simulink model "SNN_circuit11"  (R2021a)
settings: Solver=FixedStepAuto  StartTime=0.0  StopTime=50  FixedStep=1e-3  RelTol=1e-3
values from neighbouring files (symbols this model uses):
  l = 100e-6    (= 0.0001)    [SNN_run_main11.m]    (also in SNN_run_main22.m; SNN_run_main33.m)
libraries: fl_lib x57, nesl_utility x20, ee_lib x5
(part 1 of 2)
settings Model: Creator=yeeyoung  LastModifiedBy=yangy
settings SolverCC: ZeroCrossAlgorithm=Adaptive  AlgebraicLoopSolver=TrustRegion  DecoupledContinuousIntegration=on  MinimalZcImpactIntegration=on
settings DebuggingCC: SFMachineParentedDataDiag=warning
settings SimscapeCC: SimscapeLogType=all  SimscapeLogSimulationStatistics=on  SimscapeLogName=SNN_circuit1  SimscapeLogDataHistory=35000

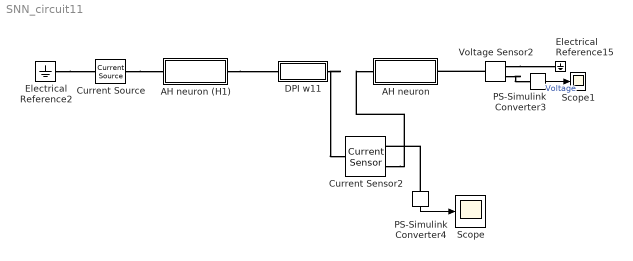
== system SNN_circuit11 ==
  AH neuron : Subsystem
  AH neuron (H1) : Subsystem
  Current Sensor2 : fl_lib/Electrical/Electrical Sensors/Current Sensor
  Current Source : ee_lib/Sources/Current Source  dc_current=Iin1 nA  ac_current=0 nA  ac_shift=0 rad  ac_frequency=60 Hz  noise_mode=0  PSD=0 A^2/Hz  repeatability=1  auto_seed=703320810  user_seed=0  sample_time=1e-3 s  i_specify=off  i_priority=None  i=0 A  i_nominal_specify=off  i_nominal_unit=A  i_nominal_value=1  v_specify=off  v_priority=None  v=0 V  v_nominal_specify=off  v_nominal_unit=V  v_nominal_value=1
      settings: SourceProductBaseCode=PS
  DPI w11 : Subsystem
  Electrical Reference15 : fl_lib/Electrical/Electrical Elements/Electrical Reference
  Electrical Reference2 : fl_lib/Electrical/Electrical Elements/Electrical Reference
  PS-Simulink Converter3 : nesl_utility/PS-Simulink Converter  PhysicalDomain=network_engine_domain  SubClassName=ps_output  LeftPortType=input  RightPortType=output  PseudoPeriodic=off  Frequencies=[]  Unit=1  AffineConversion=off
      settings: SourceProductBaseCode=PW,SS
  PS-Simulink Converter4 : nesl_utility/PS-Simulink Converter  PhysicalDomain=network_engine_domain  SubClassName=ps_output  LeftPortType=input  RightPortType=output  PseudoPeriodic=off  Frequencies=[]  Unit=1  AffineConversion=off
      settings: SourceProductBaseCode=PW,SS
  Scope : Scope
  Scope1 : Scope
  Voltage Sensor2 : fl_lib/Electrical/Electrical Sensors/Voltage Sensor
  wires:
  PS-Simulink Converter3/1 -> Scope1/1  "Voltage"
  PS-Simulink Converter4/1 -> Scope/1
  connections:
  AH neuron (H1)/RConn1 -- DPI w11/LConn1
  Voltage Sensor2/LConn1 -- AH neuron/RConn1
  Current Source/LConn1 -- AH neuron (H1)/LConn1
  Voltage Sensor2/RConn2 -- Electrical Reference15/LConn1
  Voltage Sensor2/RConn1 -- PS-Simulink Converter3/LConn1
  Electrical Reference2/LConn1 -- Current Source/RConn1
  PS-Simulink Converter4/LConn1 -- Current Sensor2/RConn1
  DPI w11/RConn1 -- Current Sensor2/LConn1
  Current Sensor2/RConn2 -- AH neuron/LConn1

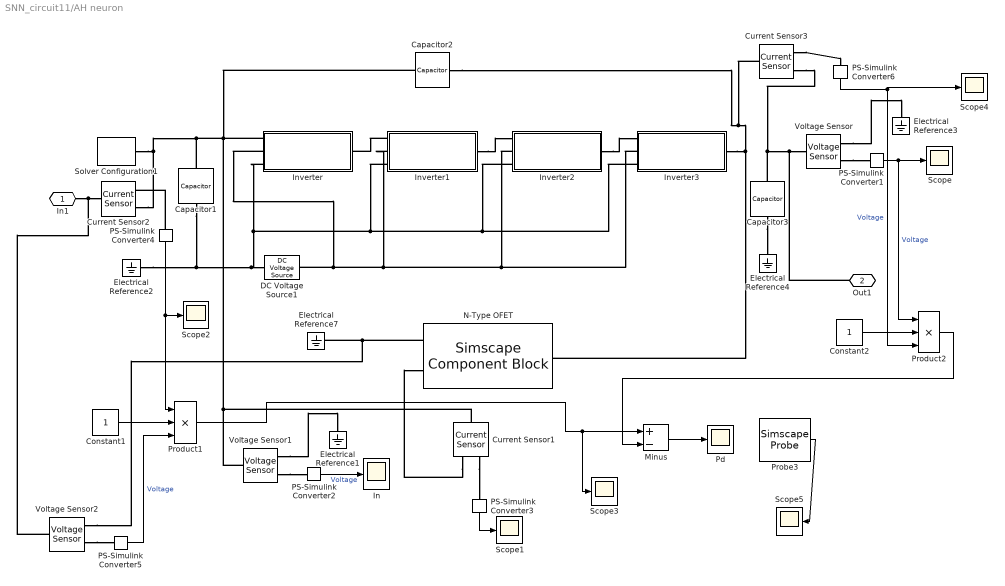
== system SNN_circuit11/AH neuron ==
  Capacitor1 : ee_lib/Passive/Capacitor  cap_option=0  c=Cmem nF  Cvec=[1e-05, 1e-06] F  Vvec=[0, 10] V  CV_table_symmetry=1  f_vec=[1, 10] kHz  DFext_vec=[.8, 1.2]  C_tol=5  enable_C_tol=0  tol_distribution=1  nSigma=4  r=1e-6 Ohm  g=0 1/Ohm  averaging_period=0 s  enable_operating_limits=0  operating_limit_action=2  max_working_voltage_range=[-25, 25] V  power_rating=1 W  enable_faults=0  fault_action=1  Cscale_faulted=100  R_faulted=1e-3 Ohm  G_faulted=0 1/Ohm  tau_fault=1e-3 s  enable_temporal_fault=0  t_fault=1 s  enable_behavioral_fault=0  max_permissible_voltage_range=[-100, 100] V  t_fail_on_voltage=1 s  i_specify=off  i_priority=None  i=0 A  i_nominal_specify=off  i_nominal_unit=A  i_nominal_value=1  v_specify=off  v_priority=None  v=0 V  v_nominal_specify=off  v_nominal_unit=V  v_nominal_value=1  vc_specify=off  vc_priority=High  vc=0 V  vc_nominal_specify=off  vc_nominal_unit=V  vc_nominal_value=1
  Capacitor2 : ee_lib/Passive/Capacitor  cap_option=0  c=Cfb nF  Cvec=[1e-05, 1e-06] F  Vvec=[0, 10] V  CV_table_symmetry=1  f_vec=[1, 10] kHz  DFext_vec=[.8, 1.2]  C_tol=5  enable_C_tol=0  tol_distribution=1  nSigma=4  r=1e-6 Ohm  g=0 1/Ohm  averaging_period=0 s  enable_operating_limits=0  operating_limit_action=2  max_working_voltage_range=[-25, 25] V  power_rating=1 W  enable_faults=0  fault_action=1  Cscale_faulted=100  R_faulted=1e-3 Ohm  G_faulted=0 1/Ohm  tau_fault=1e-3 s  enable_temporal_fault=0  t_fault=1 s  enable_behavioral_fault=0  max_permissible_voltage_range=[-100, 100] V  t_fail_on_voltage=1 s  i_specify=off  i_priority=None  i=0 A  i_nominal_specify=off  i_nominal_unit=A  i_nominal_value=1  v_specify=off  v_priority=None  v=0 V  v_nominal_specify=off  v_nominal_unit=V  v_nominal_value=1  vc_specify=off  vc_priority=High  vc=0 V  vc_nominal_specify=off  vc_nominal_unit=V  vc_nominal_value=1
  Capacitor3 : ee_lib/Passive/Capacitor  cap_option=0  c=Cload nF  Cvec=[1e-05, 1e-06] F  Vvec=[0, 10] V  CV_table_symmetry=1  f_vec=[1, 10] kHz  DFext_vec=[.8, 1.2]  C_tol=5  enable_C_tol=0  tol_distribution=1  nSigma=4  r=1e-6 Ohm  g=0 1/Ohm  averaging_period=0 s  enable_operating_limits=0  operating_limit_action=2  max_working_voltage_range=[-25, 25] V  power_rating=1 W  enable_faults=0  fault_action=1  Cscale_faulted=100  R_faulted=1e-3 Ohm  G_faulted=0 1/Ohm  tau_fault=1e-3 s  enable_temporal_fault=0  t_fault=1 s  enable_behavioral_fault=0  max_permissible_voltage_range=[-100, 100] V  t_fail_on_voltage=1 s  i_specify=off  i_priority=None  i=0 A  i_nominal_specify=off  i_nominal_unit=A  i_nominal_value=1  v_specify=off  v_priority=None  v=0 V  v_nominal_specify=off  v_nominal_unit=V  v_nominal_value=1  vc_specify=off  vc_priority=High  vc=0 V  vc_nominal_specify=off  vc_nominal_unit=V  vc_nominal_value=1
  Constant1 : Constant
  Constant2 : Constant
  Current Sensor1 : fl_lib/Electrical/Electrical Sensors/Current Sensor
  Current Sensor2 : fl_lib/Electrical/Electrical Sensors/Current Sensor
  Current Sensor3 : fl_lib/Electrical/Electrical Sensors/Current Sensor
  DC Voltage Source1 : fl_lib/Electrical/Electrical Sources/DC Voltage Source  v0=Vdd_soma V
  Electrical Reference{1..4,7} (5 alike) : fl_lib/Electrical/Electrical Elements/Electrical Reference
  In : Scope
  Inverter : Subsystem
  Inverter1 : Subsystem
  Inverter2 : Subsystem
  Inverter3 : Subsystem
  Minus : Sum  Inputs=+-
  N-Type OFET : SimscapeComponentBlock  SourceFile=N_Marinov_OFET  ComponentPath=N_Marinov_OFET  ComponentVariants=N_Marinov_OFET  ComponentVariantNames=N_Marinov_OFET  ClassName=N_Marinov_OFET  SchemaVersion=1  Gamma=gama_n  Lambda=landa_n  Vbb=Vbb_n  Vss=Vss_n  aaa=aaa_n  bbb=bbb_n  ccc=ccc_n  Mu0=mu0_n  Vt=Vt_n V  Cox=ci  W=W_n  L=l  i_specify=off  i_priority=None  i=0 A  i_nominal_specify=off  i_nominal_unit=A  i_nominal_value=1  Vgs_specify=off  Vgs_priority=None  Vgs=0 V  Vgs_nominal_specify=off  Vgs_nominal_unit=V  Vgs_nominal_value=1  Vds_specify=off  Vds_priority=None  Vds=0 V  Vds_nominal_specify=off  Vds_nominal_unit=V  Vds_nominal_value=1  Power_specify=off  Power_priority=None  Power=0 W  Power_nominal_specify=off  Power_nominal_unit=W  Power_nominal_value=1
      settings: CopyFcn=simscape.engine.sli.internal.componentblockcallback(gcbh,'COPY')  PreCopyFcn=simscape.engine.sli.internal.componentblockcallback(gcbh,'PRECOPY')  PreDeleteFcn=simscape.engine.sli.internal.componentblockcallback(gcbh,'PREDELETE')  InternalSimscapePortConfiguration="{\"Bottom\":[],\"Left\":[{\"id\":\"g\",\"label\":\"Gate\",\"type\":\"foundation.electrical.electrical\"}],\"Right\":[{\"id\":\"d\",\"label\":\"Drain\",\"type\":\"foundation.electrical.electrical\"},{\"id\":\"s\",\"label\":\"Source\",\"type\":\"foundation.electrical.electrical\"}],\"Top\":[]}"
      mask Type: Marinov OFET
  PS-Simulink Converter{1..6} (6 alike) : nesl_utility/PS-Simulink Converter  PhysicalDomain=network_engine_domain  SubClassName=ps_output  LeftPortType=input  RightPortType=output  PseudoPeriodic=off  Frequencies=[]  Unit=1  AffineConversion=off
      settings: SourceProductBaseCode=PW,SS
  Pd : Scope
  Probe3 : SimscapeProbe  BoundBlock=43  Variables={Power}
  Product1 : Product  Inputs=3
  Product2 : Product  Inputs=3
  Scope{,1..5} (6 alike) : Scope
  Solver Configuration1 : nesl_utility/Solver Configuration  PhysicalDomain=network_engine_domain  SubClassName=solver  LeftPortType=input  RightPortType=generic  Tones=[]  Harmonics=[]  SimulateNoise=off  Profile=off  UseLocalSampling=off  EnableSwitchedLinearOptims=on  FrequencyDomain=off  UseCCode=off  RelTol=0.001  AbsTol=1e-06  MinStep=1e-09  ToWorkspace=off  RevertToSquareIcSolve=off  NumHomotopyIterations=100  PhasorMode=off  PhasorModeNumHarmonics=1  DoDC=off  ResidualTolerance=1e-9  UseLocalSolver=off  LocalSolverChoice=NE_BACKWARD_EULER_ADVANCER  LocalSolverSampleTime=0.001  DoFixedCost=off  MaxNonlinIter=3  MaxModeIter=2  ComputeImpulses=off  ImpulseIterations=2  LinearAlgebra=auto  EquationFormulation=NE_TIME_EF  DelaysMemoryBudget=1024  AutomaticFiltering=off  FilteringTimeConstant=0.001  PartitionStorageMethod=AS_NEEDED  PartitionMemoryBudget=1024  PartitionMethod=ROBUST
      settings: SourceProductBaseCode=PW,SS
  Voltage Sensor : fl_lib/Electrical/Electrical Sensors/Voltage Sensor
  Voltage Sensor1 : fl_lib/Electrical/Electrical Sensors/Voltage Sensor
  Voltage Sensor2 : fl_lib/Electrical/Electrical Sensors/Voltage Sensor
  In1 : PMIOPort  Side=Left
  Out1 : PMIOPort  Port=2  Side=Right
  wires:
  PS-Simulink Converter2/1 -> In/1  "Voltage"
  PS-Simulink Converter1/1 -> Product2/1, Scope/1  "Voltage"
  PS-Simulink Converter3/1 -> Scope1/1
  PS-Simulink Converter4/1 -> Product1/1, Scope2/1
  Constant1/1 -> Product1/2
  PS-Simulink Converter5/1 -> Product1/3  "Voltage"
  Product1/1 -> Scope3/1, Minus/1
  PS-Simulink Converter6/1 -> Scope4/1, Product2/3  "Voltage"
  Constant2/1 -> Product2/2
  Product2/1 -> Minus/2
  Minus/1 -> Pd/1
  Probe3/1 -> Scope5/1
  connections:
  Inverter2/LConn3 -- Inverter3/LConn3 -- Capacitor1/RConn1 -- Electrical Reference2/LConn1 -- DC Voltage Source1/RConn1 -- Inverter/LConn3 -- Inverter1/LConn3
  Inverter2/LConn2 -- Inverter1/LConn2 -- Inverter/LConn2 -- DC Voltage Source1/LConn1 -- Inverter3/LConn2
  Out1/RConn1 -- Capacitor3/LConn1 -- Current Sensor3/RConn2 -- Voltage Sensor/LConn1
  Solver Configuration1/RConn1 -- Current Sensor2/RConn2 -- Capacitor1/LConn1 -- Capacitor2/RConn1 -- Current Sensor1/LConn1 -- Voltage Sensor1/LConn1 -- Inverter/LConn1
  Inverter1/LConn1 -- Inverter/RConn1
  Inverter1/RConn1 -- Inverter2/LConn1
  N-Type OFET/RConn2 -- Voltage Sensor2/RConn2 -- Electrical Reference7/LConn1
  Voltage Sensor1/RConn1 -- PS-Simulink Converter2/LConn1
  Voltage Sensor/RConn1 -- PS-Simulink Converter1/LConn1
  Voltage Sensor/RConn2 -- Electrical Reference3/LConn1
  Voltage Sensor1/RConn2 -- Electrical Reference1/LConn1
  Inverter2/RConn1 -- Inverter3/LConn1
  Current Sensor1/RConn2 -- N-Type OFET/RConn1
  Current Sensor1/RConn1 -- PS-Simulink Converter3/LConn1
  Capacitor3/RConn1 -- Electrical Reference4/LConn1
  In1/RConn1 -- Voltage Sensor2/LConn1 -- Current Sensor2/LConn1
  PS-Simulink Converter4/LConn1 -- Current Sensor2/RConn1
  Voltage Sensor2/RConn1 -- PS-Simulink Converter5/LConn1
  Capacitor2/LConn1 -- Current Sensor3/LConn1 -- Inverter3/RConn1 -- N-Type OFET/LConn1
  Current Sensor3/RConn1 -- PS-Simulink Converter6/LConn1

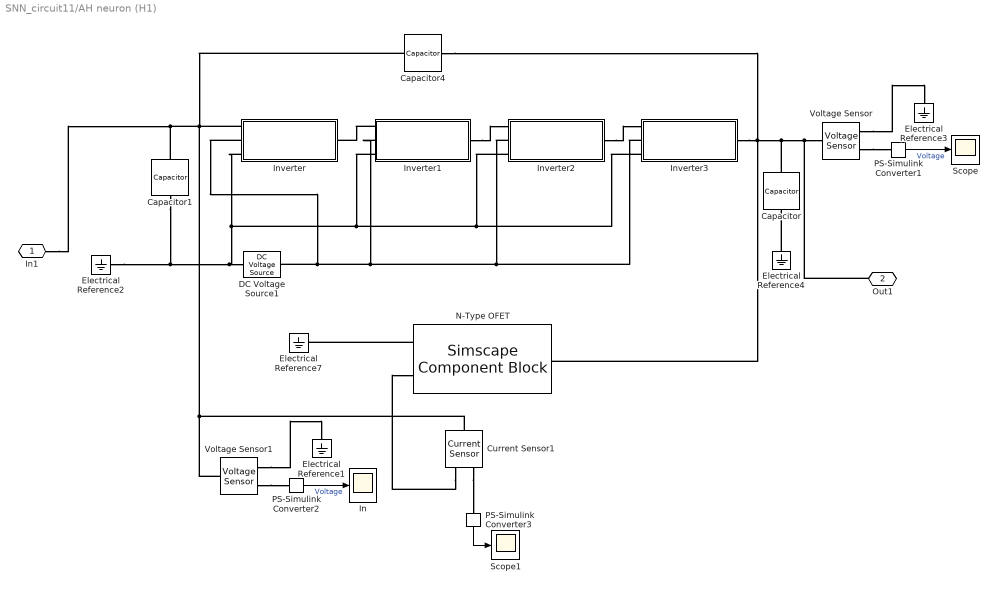
== system SNN_circuit11/AH neuron (H1) ==
  Capacitor : fl_lib/Electrical/Electrical Elements/Capacitor  c=Cload nF  r=1e-6 Ohm  g=0 1/Ohm  i_specify=off  i_priority=None  i=0 A  i_nominal_specify=off  i_nominal_unit=A  i_nominal_value=1  v_specify=off  v_priority=None  v=0 V  v_nominal_specify=off  v_nominal_unit=V  v_nominal_value=1  vc_specify=off  vc_priority=High  vc=0 V  vc_nominal_specify=off  vc_nominal_unit=V  vc_nominal_value=1
  Capacitor1 : ee_lib/Passive/Capacitor  cap_option=0  c=Cmem nF  Cvec=[1e-05, 1e-06] F  Vvec=[0, 10] V  CV_table_symmetry=1  f_vec=[1, 10] kHz  DFext_vec=[.8, 1.2]  C_tol=5  enable_C_tol=0  tol_distribution=1  nSigma=4  r=1e-6 Ohm  g=0 1/Ohm  averaging_period=0 s  enable_operating_limits=0  operating_limit_action=2  max_working_voltage_range=[-25, 25] V  power_rating=1 W  enable_faults=0  fault_action=1  Cscale_faulted=100  R_faulted=1e-3 Ohm  G_faulted=0 1/Ohm  tau_fault=1e-3 s  enable_temporal_fault=0  t_fault=1 s  enable_behavioral_fault=0  max_permissible_voltage_range=[-100, 100] V  t_fail_on_voltage=1 s  i_specify=off  i_priority=None  i=0 A  i_nominal_specify=off  i_nominal_unit=A  i_nominal_value=1  v_specify=off  v_priority=None  v=0 V  v_nominal_specify=off  v_nominal_unit=V  v_nominal_value=1  vc_specify=off  vc_priority=High  vc=0 V  vc_nominal_specify=off  vc_nominal_unit=V  vc_nominal_value=1
  Capacitor4 : fl_lib/Electrical/Electrical Elements/Capacitor  c=Cfb nF  r=1e-6 Ohm  g=0 1/Ohm  i_specify=off  i_priority=None  i=0 A  i_nominal_specify=off  i_nominal_unit=A  i_nominal_value=1  v_specify=off  v_priority=None  v=0 V  v_nominal_specify=off  v_nominal_unit=V  v_nominal_value=1  vc_specify=off  vc_priority=High  vc=0 V  vc_nominal_specify=off  vc_nominal_unit=V  vc_nominal_value=1
  Current Sensor1 : fl_lib/Electrical/Electrical Sensors/Current Sensor
  DC Voltage Source1 : fl_lib/Electrical/Electrical Sources/DC Voltage Source  v0=Vdd_soma V
  Electrical Reference{1..4,7} (5 alike) : fl_lib/Electrical/Electrical Elements/Electrical Reference
  In : Scope
  Inverter : Subsystem
  Inverter1 : Subsystem
  Inverter2 : Subsystem
  Inverter3 : Subsystem
  N-Type OFET : SimscapeComponentBlock  SourceFile=N_Marinov_OFET  ComponentPath=N_Marinov_OFET  ComponentVariants=N_Marinov_OFET  ComponentVariantNames=N_Marinov_OFET  ClassName=N_Marinov_OFET  SchemaVersion=1  Gamma=gama_n  Lambda=landa_n  Vbb=Vbb_n  Vss=Vss_n  aaa=aaa_n  bbb=bbb_n  ccc=ccc_n  Mu0=mu0_n  Vt=Vt_n V  Cox=ci  W=W_n  L=l  i_specify=off  i_priority=None  i=0 A  i_nominal_specify=off  i_nominal_unit=A  i_nominal_value=1  Vgs_specify=off  Vgs_priority=None  Vgs=0 V  Vgs_nominal_specify=off  Vgs_nominal_unit=V  Vgs_nominal_value=1  Vds_specify=off  Vds_priority=None  Vds=0 V  Vds_nominal_specify=off  Vds_nominal_unit=V  Vds_nominal_value=1  Power_specify=off  Power_priority=None  Power=0 W  Power_nominal_specify=off  Power_nominal_unit=W  Power_nominal_value=1
      settings: CopyFcn=simscape.engine.sli.internal.componentblockcallback(gcbh,'COPY')  PreCopyFcn=simscape.engine.sli.internal.componentblockcallback(gcbh,'PRECOPY')  PreDeleteFcn=simscape.engine.sli.internal.componentblockcallback(gcbh,'PREDELETE')  InternalSimscapePortConfiguration="{\"Bottom\":[],\"Left\":[{\"id\":\"g\",\"label\":\"Gate\",\"type\":\"foundation.electrical.electrical\"}],\"Right\":[{\"id\":\"d\",\"label\":\"Drain\",\"type\":\"foundation.electrical.electrical\"},{\"id\":\"s\",\"label\":\"Source\",\"type\":\"foundation.electrical.electrical\"}],\"Top\":[]}"
      mask Type: Marinov OFET
  PS-Simulink Converter1 : nesl_utility/PS-Simulink Converter  PhysicalDomain=network_engine_domain  SubClassName=ps_output  LeftPortType=input  RightPortType=output  PseudoPeriodic=off  Frequencies=[]  Unit=1  AffineConversion=off
      settings: SourceProductBaseCode=PW,SS
  PS-Simulink Converter2 : nesl_utility/PS-Simulink Converter  PhysicalDomain=network_engine_domain  SubClassName=ps_output  LeftPortType=input  RightPortType=output  PseudoPeriodic=off  Frequencies=[]  Unit=1  AffineConversion=off
      settings: SourceProductBaseCode=PW,SS
  PS-Simulink Converter3 : nesl_utility/PS-Simulink Converter  PhysicalDomain=network_engine_domain  SubClassName=ps_output  LeftPortType=input  RightPortType=output  PseudoPeriodic=off  Frequencies=[]  Unit=1  AffineConversion=off
      settings: SourceProductBaseCode=PW,SS
  Scope : Scope
  Scope1 : Scope
  Voltage Sensor : fl_lib/Electrical/Electrical Sensors/Voltage Sensor
  Voltage Sensor1 : fl_lib/Electrical/Electrical Sensors/Voltage Sensor
  In1 : PMIOPort  Side=Left
  Out1 : PMIOPort  Port=2  Side=Right
  wires:
  PS-Simulink Converter2/1 -> In/1  "Voltage"
  PS-Simulink Converter1/1 -> Scope/1  "Voltage"
  PS-Simulink Converter3/1 -> Scope1/1
  connections:
  Inverter2/LConn3 -- Inverter3/LConn3 -- Capacitor1/RConn1 -- Electrical Reference2/LConn1 -- DC Voltage Source1/RConn1 -- Inverter/LConn3 -- Inverter1/LConn3
  Inverter2/LConn2 -- Inverter1/LConn2 -- Inverter/LConn2 -- DC Voltage Source1/LConn1 -- Inverter3/LConn2
  Capacitor4/LConn1 -- Inverter3/RConn1 -- N-Type OFET/LConn1 -- Capacitor/LConn1 -- Out1/RConn1 -- Voltage Sensor/LConn1
  Capacitor1/LConn1 -- In1/RConn1 -- Capacitor4/RConn1 -- Current Sensor1/LConn1 -- Voltage Sensor1/LConn1 -- Inverter/LConn1
  Inverter1/LConn1 -- Inverter/RConn1
  Inverter1/RConn1 -- Inverter2/LConn1
  N-Type OFET/RConn2 -- Electrical Reference7/LConn1
  Voltage Sensor1/RConn1 -- PS-Simulink Converter2/LConn1
  Voltage Sensor/RConn1 -- PS-Simulink Converter1/LConn1
  Voltage Sensor/RConn2 -- Electrical Reference3/LConn1
  Voltage Sensor1/RConn2 -- Electrical Reference1/LConn1
  Inverter2/RConn1 -- Inverter3/LConn1
  Current Sensor1/RConn2 -- N-Type OFET/RConn1
  Current Sensor1/RConn1 -- PS-Simulink Converter3/LConn1
  Electrical Reference4/LConn1 -- Capacitor/RConn1

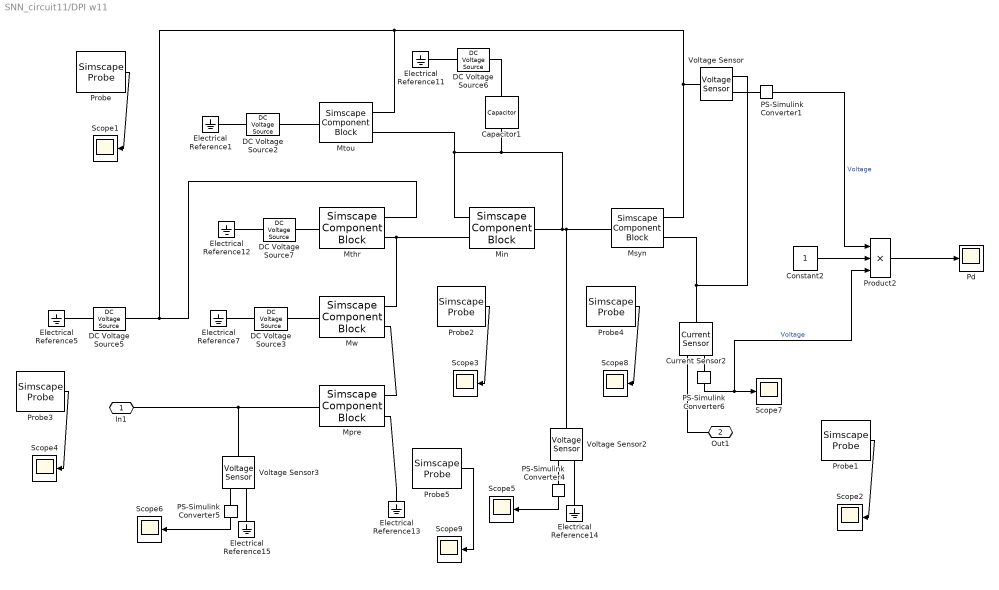
== system SNN_circuit11/DPI w11 ==
  Capacitor1 : fl_lib/Electrical/Electrical Elements/Capacitor  c=Csyn nF  r=1e-6 Ohm  g=0 1/Ohm  i_specify=off  i_priority=None  i=0 A  i_nominal_specify=off  i_nominal_unit=A  i_nominal_value=1  v_specify=off  v_priority=None  v=0 V  v_nominal_specify=off  v_nominal_unit=V  v_nominal_value=1  vc_specify=off  vc_priority=High  vc=0 V  vc_nominal_specify=off  vc_nominal_unit=V  vc_nominal_value=1
  Constant2 : Constant
  Current Sensor2 : fl_lib/Electrical/Electrical Sensors/Current Sensor
  DC Voltage Source2 : fl_lib/Electrical/Electrical Sources/DC Voltage Source  v0=Vtau V
  DC Voltage Source3 : fl_lib/Electrical/Electrical Sources/DC Voltage Source  v0=Vw V
  DC Voltage Source5 : fl_lib/Electrical/Electrical Sources/DC Voltage Source  v0=Vdd_syn V
  DC Voltage Source6 : fl_lib/Electrical/Electrical Sources/DC Voltage Source  v0=Vdd_syn V
  DC Voltage Source7 : fl_lib/Electrical/Electrical Sources/DC Voltage Source  v0=Vthr V
  Electrical Reference{1,5,7,11..15} (8 alike) : fl_lib/Electrical/Electrical Elements/Electrical Reference
  Min : SimscapeComponentBlock  SourceFile=N_Marinov_OFET  ComponentPath=N_Marinov_OFET  ComponentVariants=N_Marinov_OFET  ComponentVariantNames=N_Marinov_OFET  ClassName=N_Marinov_OFET  SchemaVersion=1  Gamma=gama_n  Lambda=landa_n  Vbb=Vbb_n  Vss=Vss_n  aaa=aaa_n  bbb=bbb_n  ccc=ccc_n  Mu0=mu0_n  Vt=Vt_n V  Cox=ci  W=W_n  L=l  i_specify=off  i_priority=None  i=0 A  i_nominal_specify=off  i_nominal_unit=A  i_nominal_value=1  Vgs_specify=off  Vgs_priority=None  Vgs=0 V  Vgs_nominal_specify=off  Vgs_nominal_unit=V  Vgs_nominal_value=1  Vds_specify=off  Vds_priority=None  Vds=0 V  Vds_nominal_specify=off  Vds_nominal_unit=V  Vds_nominal_value=1  Power_specify=off  Power_priority=None  Power=0 W  Power_nominal_specify=off  Power_nominal_unit=W  Power_nominal_value=1
      settings: CopyFcn=simscape.engine.sli.internal.componentblockcallback(gcbh,'COPY')  PreCopyFcn=simscape.engine.sli.internal.componentblockcallback(gcbh,'PRECOPY')  PreDeleteFcn=simscape.engine.sli.internal.componentblockcallback(gcbh,'PREDELETE')  InternalSimscapePortConfiguration="{\"Bottom\":[],\"Left\":[{\"id\":\"g\",\"label\":\"Gate\",\"type\":\"foundation.electrical.electrical\"}],\"Right\":[{\"id\":\"d\",\"label\":\"Drain\",\"type\":\"foundation.electrical.electrical\"},{\"id\":\"s\",\"label\":\"Source\",\"type\":\"foundation.electrical.electrical\"}],\"Top\":[]}"
      mask Type: Marinov OFET
  Mpre : SimscapeComponentBlock  SourceFile=N_Marinov_OFET  ComponentPath=N_Marinov_OFET  ComponentVariants=N_Marinov_OFET  ComponentVariantNames=N_Marinov_OFET  ClassName=N_Marinov_OFET  SchemaVersion=1  Gamma=gama_n  Lambda=landa_n  Vbb=Vbb_n  Vss=Vss_n  aaa=aaa_n  bbb=bbb_n  ccc=ccc_n  Mu0=mu0_n  Vt=Vt_n V  Cox=ci  W=W_n  L=l  i_specify=off  i_priority=None  i=0 A  i_nominal_specify=off  i_nominal_unit=A  i_nominal_value=1  Vgs_specify=off  Vgs_priority=None  Vgs=0 V  Vgs_nominal_specify=off  Vgs_nominal_unit=V  Vgs_nominal_value=1  Vds_specify=off  Vds_priority=None  Vds=0 V  Vds_nominal_specify=off  Vds_nominal_unit=V  Vds_nominal_value=1  Power_specify=off  Power_priority=None  Power=0 W  Power_nominal_specify=off  Power_nominal_unit=W  Power_nominal_value=1
      settings: CopyFcn=simscape.engine.sli.internal.componentblockcallback(gcbh,'COPY')  PreCopyFcn=simscape.engine.sli.internal.componentblockcallback(gcbh,'PRECOPY')  PreDeleteFcn=simscape.engine.sli.internal.componentblockcallback(gcbh,'PREDELETE')  InternalSimscapePortConfiguration="{\"Bottom\":[],\"Left\":[{\"id\":\"g\",\"label\":\"Gate\",\"type\":\"foundation.electrical.electrical\"}],\"Right\":[{\"id\":\"d\",\"label\":\"Drain\",\"type\":\"foundation.electrical.electrical\"},{\"id\":\"s\",\"label\":\"Source\",\"type\":\"foundation.electrical.electrical\"}],\"Top\":[]}"
      mask Type: Marinov OFET
  Msyn : SimscapeComponentBlock  SourceFile=P_Marinov_OFET  ComponentPath=P_Marinov_OFET  ComponentVariants=P_Marinov_OFET  ComponentVariantNames=P_Marinov_OFET  ClassName=P_Marinov_OFET  SchemaVersion=1  Gamma=gama_p  Lambda=landa_p  Vbb=Vbb_p  Vss=Vss_p  aaa=aaa_p  bbb=bbb_p  ccc=ccc_p  Mu0=mu0_p  Vt=Vt_p V  Cox=ci  W=W_p  L=l  i_specify=off  i_priority=None  i=0 A  i_nominal_specify=off  i_nominal_unit=A  i_nominal_value=1  Vsg_specify=off  Vsg_priority=None  Vsg=0 V  Vsg_nominal_specify=off  Vsg_nominal_unit=V  Vsg_nominal_value=1  Vsd_specify=off  Vsd_priority=None  Vsd=0 V  Vsd_nominal_specify=off  Vsd_nominal_unit=V  Vsd_nominal_value=1  Power_specify=off  Power_priority=None  Power=0 W  Power_nominal_specify=off  Power_nominal_unit=W  Power_nominal_value=1
      settings: CopyFcn=simscape.engine.sli.internal.componentblockcallback(gcbh,'COPY')  PreCopyFcn=simscape.engine.sli.internal.componentblockcallback(gcbh,'PRECOPY')  PreDeleteFcn=simscape.engine.sli.internal.componentblockcallback(gcbh,'PREDELETE')  InternalSimscapePortConfiguration="{\"Bottom\":[],\"Left\":[{\"id\":\"g\",\"label\":\"Gate\",\"type\":\"foundation.electrical.electrical\"}],\"Right\":[{\"id\":\"s\",\"label\":\"Source\",\"type\":\"foundation.electrical.electrical\"},{\"id\":\"d\",\"label\":\"Drain\",\"type\":\"foundation.electrical.electrical\"}],\"Top\":[]}"
      mask Type: Marinov OFET
  Mthr : SimscapeComponentBlock  SourceFile=N_Marinov_OFET  ComponentPath=N_Marinov_OFET  ComponentVariants=N_Marinov_OFET  ComponentVariantNames=N_Marinov_OFET  ClassName=N_Marinov_OFET  SchemaVersion=1  Gamma=gama_n  Lambda=landa_n  Vbb=Vbb_n  Vss=Vss_n  aaa=aaa_n  bbb=bbb_n  ccc=ccc_n  Mu0=mu0_n  Vt=Vt_n V  Cox=ci  W=W_n  L=l  i_specify=off  i_priority=None  i=0 A  i_nominal_specify=off  i_nominal_unit=A  i_nominal_value=1  Vgs_specify=off  Vgs_priority=None  Vgs=0 V  Vgs_nominal_specify=off  Vgs_nominal_unit=V  Vgs_nominal_value=1  Vds_specify=off  Vds_priority=None  Vds=0 V  Vds_nominal_specify=off  Vds_nominal_unit=V  Vds_nominal_value=1  Power_specify=off  Power_priority=None  Power=0 W  Power_nominal_specify=off  Power_nominal_unit=W  Power_nominal_value=1
      settings: CopyFcn=simscape.engine.sli.internal.componentblockcallback(gcbh,'COPY')  PreCopyFcn=simscape.engine.sli.internal.componentblockcallback(gcbh,'PRECOPY')  PreDeleteFcn=simscape.engine.sli.internal.componentblockcallback(gcbh,'PREDELETE')  InternalSimscapePortConfiguration="{\"Bottom\":[],\"Left\":[{\"id\":\"g\",\"label\":\"Gate\",\"type\":\"foundation.electrical.electrical\"}],\"Right\":[{\"id\":\"d\",\"label\":\"Drain\",\"type\":\"foundation.electrical.electrical\"},{\"id\":\"s\",\"label\":\"Source\",\"type\":\"foundation.electrical.electrical\"}],\"Top\":[]}"
      mask Type: Marinov OFET
  Mtou : SimscapeComponentBlock  SourceFile=P_Marinov_OFET  ComponentPath=P_Marinov_OFET  ComponentVariants=P_Marinov_OFET  ComponentVariantNames=P_Marinov_OFET  ClassName=P_Marinov_OFET  SchemaVersion=1  Gamma=gama_p  Lambda=landa_p  Vbb=Vbb_p  Vss=Vss_p  aaa=aaa_p  bbb=bbb_p  ccc=ccc_p  Mu0=mu0_p  Vt=Vt_p V  Cox=ci  W=W_p  L=l  i_specify=off  i_priority=None  i=0 A  i_nominal_specify=off  i_nominal_unit=A  i_nominal_value=1  Vsg_specify=off  Vsg_priority=None  Vsg=0 V  Vsg_nominal_specify=off  Vsg_nominal_unit=V  Vsg_nominal_value=1  Vsd_specify=off  Vsd_priority=None  Vsd=0 V  Vsd_nominal_specify=off  Vsd_nominal_unit=V  Vsd_nominal_value=1  Power_specify=off  Power_priority=None  Power=0 W  Power_nominal_specify=off  Power_nominal_unit=W  Power_nominal_value=1
      settings: CopyFcn=simscape.engine.sli.internal.componentblockcallback(gcbh,'COPY')  PreCopyFcn=simscape.engine.sli.internal.componentblockcallback(gcbh,'PRECOPY')  PreDeleteFcn=simscape.engine.sli.internal.componentblockcallback(gcbh,'PREDELETE')  InternalSimscapePortConfiguration="{\"Bottom\":[],\"Left\":[{\"id\":\"g\",\"label\":\"Gate\",\"type\":\"foundation.electrical.electrical\"}],\"Right\":[{\"id\":\"s\",\"label\":\"Source\",\"type\":\"foundation.electrical.electrical\"},{\"id\":\"d\",\"label\":\"Drain\",\"type\":\"foundation.electrical.electrical\"}],\"Top\":[]}"
      mask Type: Marinov OFET
  Mw : SimscapeComponentBlock  SourceFile=N_Marinov_OFET  ComponentPath=N_Marinov_OFET  ComponentVariants=N_Marinov_OFET  ComponentVariantNames=N_Marinov_OFET  ClassName=N_Marinov_OFET  SchemaVersion=1  Gamma=gama_n  Lambda=landa_n  Vbb=Vbb_n  Vss=Vss_n  aaa=aaa_n  bbb=bbb_n  ccc=ccc_n  Mu0=mu0_n  Vt=Vt_n V  Cox=ci  W=W_n  L=l  i_specify=off  i_priority=None  i=0 A  i_nominal_specify=off  i_nominal_unit=A  i_nominal_value=1  Vgs_specify=off  Vgs_priority=None  Vgs=0 V  Vgs_nominal_specify=off  Vgs_nominal_unit=V  Vgs_nominal_value=1  Vds_specify=off  Vds_priority=None  Vds=0 V  Vds_nominal_specify=off  Vds_nominal_unit=V  Vds_nominal_value=1  Power_specify=off  Power_priority=None  Power=0 W  Power_nominal_specify=off  Power_nominal_unit=W  Power_nominal_value=1
      settings: CopyFcn=simscape.engine.sli.internal.componentblockcallback(gcbh,'COPY')  PreCopyFcn=simscape.engine.sli.internal.componentblockcallback(gcbh,'PRECOPY')  PreDeleteFcn=simscape.engine.sli.internal.componentblockcallback(gcbh,'PREDELETE')  InternalSimscapePortConfiguration="{\"Bottom\":[],\"Left\":[{\"id\":\"g\",\"label\":\"Gate\",\"type\":\"foundation.electrical.electrical\"}],\"Right\":[{\"id\":\"d\",\"label\":\"Drain\",\"type\":\"foundation.electrical.electrical\"},{\"id\":\"s\",\"label\":\"Source\",\"type\":\"foundation.electrical.electrical\"}],\"Top\":[]}"
      mask Type: Marinov OFET
  PS-Simulink Converter{1,4..6} (4 alike) : nesl_utility/PS-Simulink Converter  PhysicalDomain=network_engine_domain  SubClassName=ps_output  LeftPortType=input  RightPortType=output  PseudoPeriodic=off  Frequencies=[]  Unit=1  AffineConversion=off
      settings: SourceProductBaseCode=PW,SS
  Pd : Scope
  Probe : SimscapeProbe  BoundBlock=1208  Variables={Power}
  Probe1 : SimscapeProbe  BoundBlock=1206  Variables={Power}
  Probe2 : SimscapeProbe  BoundBlock=1207  Variables={Power}
  Probe3 : SimscapeProbe  BoundBlock=1209  Variables={Power}
  Probe4 : SimscapeProbe  BoundBlock=1204  Variables={Power}
  Probe5 : SimscapeProbe  BoundBlock=1205  Variables={Power}
  Product2 : Product  Inputs=3
  Scope{1..9} (9 alike) : Scope
  Voltage Sensor : fl_lib/Electrical/Electrical Sensors/Voltage Sensor
  Voltage Sensor2 : fl_lib/Electrical/Electrical Sensors/Voltage Sensor
  Voltage Sensor3 : fl_lib/Electrical/Electrical Sensors/Voltage Sensor
  In1 : PMIOPort  Side=Left
  Out1 : PMIOPort  Port=2  Side=Right
  wires:
  PS-Simulink Converter5/1 -> Scope6/1
  PS-Simulink Converter4/1 -> Scope5/1
  Constant2/1 -> Product2/2
  PS-Simulink Converter6/1 -> Product2/3, Scope7/1  "Voltage"
  Product2/1 -> Pd/1
  PS-Simulink Converter1/1 -> Product2/1  "Voltage"
  Probe/1 -> Scope1/1
  Probe1/1 -> Scope2/1
  Probe2/1 -> Scope3/1
  Probe3/1 -> Scope4/1
  Probe4/1 -> Scope8/1
  Probe5/1 -> Scope9/1
  connections:
  Mtou/RConn1 -- DC Voltage Source5/LConn1 -- Mthr/RConn1 -- Voltage Sensor/LConn1 -- Msyn/RConn1
  Current Sensor2/RConn2 -- Out1/RConn1
  Min/LConn1 -- Capacitor1/RConn1 -- Min/RConn1 -- Mtou/RConn2 -- Msyn/LConn1 -- Voltage Sensor2/LConn1
  Mthr/RConn2 -- Mw/RConn1 -- Min/RConn2
  Mpre/RConn1 -- Mw/RConn2
  Mpre/LConn1 -- In1/RConn1 -- Voltage Sensor3/LConn1
  Electrical Reference11/LConn1 -- DC Voltage Source6/RConn1
  PS-Simulink Converter4/LConn1 -- Voltage Sensor2/RConn1
  Electrical Reference5/LConn1 -- DC Voltage Source5/RConn1
  Electrical Reference7/LConn1 -- DC Voltage Source3/RConn1
  DC Voltage Source7/LConn1 -- Mthr/LConn1
  DC Voltage Source2/LConn1 -- Mtou/LConn1
  Electrical Reference12/LConn1 -- DC Voltage Source7/RConn1
  Electrical Reference15/LConn1 -- Voltage Sensor3/RConn2
  Electrical Reference14/LConn1 -- Voltage Sensor2/RConn2
  Current Sensor2/RConn1 -- PS-Simulink Converter6/LConn1
  Electrical Reference13/LConn1 -- Mpre/RConn2
  Current Sensor2/LConn1 -- Voltage Sensor/RConn2 -- Msyn/RConn2
  Electrical Reference1/LConn1 -- DC Voltage Source2/RConn1
  DC Voltage Source3/LConn1 -- Mw/LConn1
  PS-Simulink Converter5/LConn1 -- Voltage Sensor3/RConn1
  DC Voltage Source6/LConn1 -- Capacitor1/LConn1
  Voltage Sensor/RConn1 -- PS-Simulink Converter1/LConn1

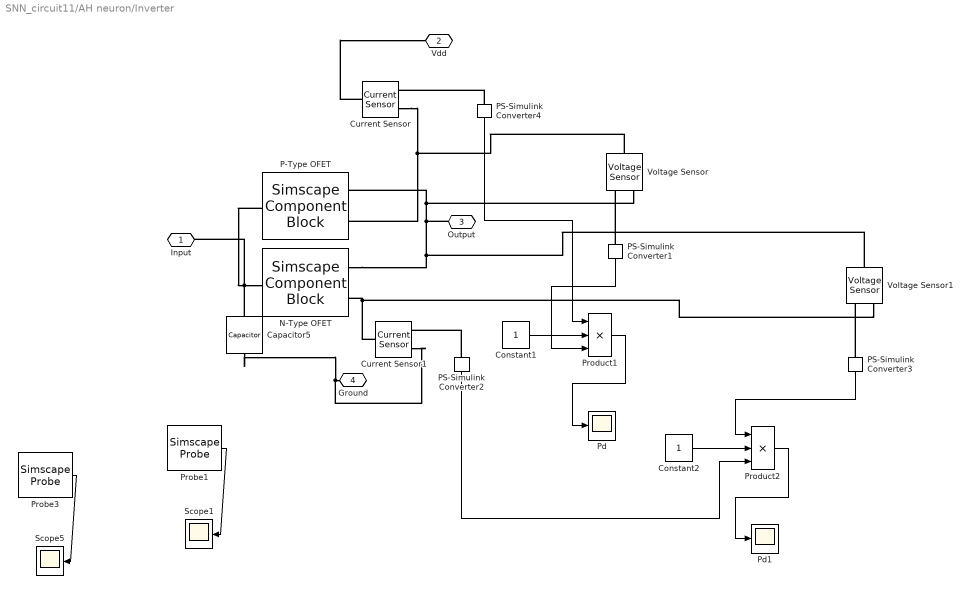
== system SNN_circuit11/AH neuron/Inverter ==
  Capacitor5 : fl_lib/Electrical/Electrical Elements/Capacitor  c=Cgs nF  r=1e-12 Ohm  g=0 1/Ohm  i_specify=off  i_priority=None  i=0 A  i_nominal_specify=off  i_nominal_unit=A  i_nominal_value=1  v_specify=off  v_priority=None  v=0 V  v_nominal_specify=off  v_nominal_unit=V  v_nominal_value=1  vc_specify=off  vc_priority=High  vc=0 V  vc_nominal_specify=off  vc_nominal_unit=V  vc_nominal_value=1
  Constant1 : Constant
  Constant2 : Constant
  Current Sensor : fl_lib/Electrical/Electrical Sensors/Current Sensor
  Current Sensor1 : fl_lib/Electrical/Electrical Sensors/Current Sensor
  N-Type OFET : SimscapeComponentBlock  SourceFile=N_Marinov_OFET  ComponentPath=N_Marinov_OFET  ComponentVariants=N_Marinov_OFET  ComponentVariantNames=N_Marinov_OFET  ClassName=N_Marinov_OFET  SchemaVersion=1  Gamma=gama_n  Lambda=landa_n  Vbb=Vbb_n  Vss=Vss_n  aaa=aaa_n  bbb=bbb_n  ccc=ccc_n  Mu0=mu0_n  Vt=Vt_n V  Cox=ci  W=W_n  L=l  i_specify=off  i_priority=None  i=0 A  i_nominal_specify=off  i_nominal_unit=A  i_nominal_value=1  Vgs_specify=off  Vgs_priority=None  Vgs=0 V  Vgs_nominal_specify=off  Vgs_nominal_unit=V  Vgs_nominal_value=1  Vds_specify=off  Vds_priority=None  Vds=0 V  Vds_nominal_specify=off  Vds_nominal_unit=V  Vds_nominal_value=1  Power_specify=off  Power_priority=None  Power=0 W  Power_nominal_specify=off  Power_nominal_unit=W  Power_nominal_value=1
      settings: CopyFcn=simscape.engine.sli.internal.componentblockcallback(gcbh,'COPY')  PreCopyFcn=simscape.engine.sli.internal.componentblockcallback(gcbh,'PRECOPY')  PreDeleteFcn=simscape.engine.sli.internal.componentblockcallback(gcbh,'PREDELETE')  InternalSimscapePortConfiguration="{\"Bottom\":[],\"Left\":[{\"id\":\"g\",\"label\":\"Gate\",\"type\":\"foundation.electrical.electrical\"}],\"Right\":[{\"id\":\"d\",\"label\":\"Drain\",\"type\":\"foundation.electrical.electrical\"},{\"id\":\"s\",\"label\":\"Source\",\"type\":\"foundation.electrical.electrical\"}],\"Top\":[]}"
      mask Type: Marinov OFET
  P-Type OFET : SimscapeComponentBlock  SourceFile=P_Marinov_OFET  ComponentPath=P_Marinov_OFET  ComponentVariants=P_Marinov_OFET  ComponentVariantNames=P_Marinov_OFET  ClassName=P_Marinov_OFET  SchemaVersion=1  Gamma=gama_p  Lambda=landa_p  Vbb=Vbb_p  Vss=Vss_p  aaa=aaa_p  bbb=bbb_p  ccc=ccc_p  Mu0=mu0_p  Vt=Vt_p V  Cox=ci  W=W_p  L=l  i_specify=off  i_priority=None  i=0 A  i_nominal_specify=off  i_nominal_unit=A  i_nominal_value=1  Vsg_specify=off  Vsg_priority=None  Vsg=0 V  Vsg_nominal_specify=off  Vsg_nominal_unit=V  Vsg_nominal_value=1  Vsd_specify=off  Vsd_priority=None  Vsd=0 V  Vsd_nominal_specify=off  Vsd_nominal_unit=V  Vsd_nominal_value=1  Power_specify=off  Power_priority=None  Power=0 W  Power_nominal_specify=off  Power_nominal_unit=W  Power_nominal_value=1
      settings: CopyFcn=simscape.engine.sli.internal.componentblockcallback(gcbh,'COPY')  PreCopyFcn=simscape.engine.sli.internal.componentblockcallback(gcbh,'PRECOPY')  PreDeleteFcn=simscape.engine.sli.internal.componentblockcallback(gcbh,'PREDELETE')  InternalSimscapePortConfiguration="{\"Bottom\":[],\"Left\":[{\"id\":\"g\",\"label\":\"Gate\",\"type\":\"foundation.electrical.electrical\"}],\"Right\":[{\"id\":\"s\",\"label\":\"Source\",\"type\":\"foundation.electrical.electrical\"},{\"id\":\"d\",\"label\":\"Drain\",\"type\":\"foundation.electrical.electrical\"}],\"Top\":[]}"
      mask Type: Marinov OFET
  PS-Simulink Converter{1..4} (4 alike) : nesl_utility/PS-Simulink Converter  PhysicalDomain=network_engine_domain  SubClassName=ps_output  LeftPortType=input  RightPortType=output  PseudoPeriodic=off  Frequencies=[]  Unit=1  AffineConversion=off
      settings: SourceProductBaseCode=PW,SS
  Pd : Scope
  Pd1 : Scope
  Probe1 : SimscapeProbe  BoundBlock=16  Variables={Power}
  Probe3 : SimscapeProbe  BoundBlock=17  Variables={Power}
  Product1 : Product  Inputs=3
  Product2 : Product  Inputs=3
  Scope1 : Scope
  Scope5 : Scope
  Voltage Sensor : fl_lib/Electrical/Electrical Sensors/Voltage Sensor
  Voltage Sensor1 : fl_lib/Electrical/Electrical Sensors/Voltage Sensor
  Input : PMIOPort  Side=Left
  Vdd : PMIOPort  Port=2  Side=Left
  Output : PMIOPort  Port=3  Side=Right
  Ground : PMIOPort  Port=4  Side=Left
  wires:
  PS-Simulink Converter4/1 -> Product1/1
  Constant1/1 -> Product1/2
  Product1/1 -> Pd/1
  PS-Simulink Converter1/1 -> Product1/3
  Constant2/1 -> Product2/2
  PS-Simulink Converter3/1 -> Product2/1
  Product2/1 -> Pd1/1
  PS-Simulink Converter2/1 -> Product2/3
  Probe3/1 -> Scope5/1
  Probe1/1 -> Scope1/1
  connections:
  N-Type OFET/RConn1 -- Voltage Sensor1/LConn1 -- Output/RConn1 -- Voltage Sensor/RConn2 -- P-Type OFET/RConn2
  Input/RConn1 -- P-Type OFET/LConn1 -- Capacitor5/LConn1 -- N-Type OFET/LConn1
  Capacitor5/RConn1 -- Current Sensor1/RConn2 -- Ground/RConn1
  Current Sensor/LConn1 -- Vdd/RConn1
  Current Sensor/RConn2 -- Voltage Sensor/LConn1 -- P-Type OFET/RConn1
  PS-Simulink Converter4/LConn1 -- Current Sensor/RConn1
  PS-Simulink Converter1/LConn1 -- Voltage Sensor/RConn1
  PS-Simulink Converter2/LConn1 -- Current Sensor1/RConn1
  Current Sensor1/LConn1 -- Voltage Sensor1/RConn2 -- N-Type OFET/RConn2
  PS-Simulink Converter3/LConn1 -- Voltage Sensor1/RConn1

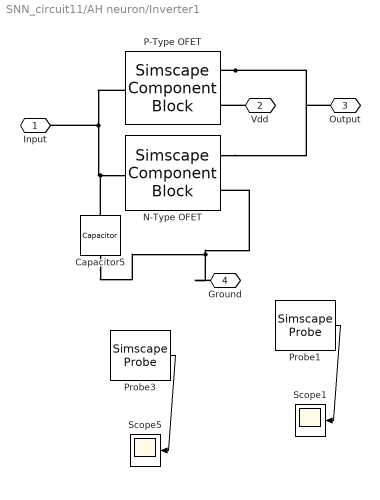
== system SNN_circuit11/AH neuron/Inverter1 ==
  Capacitor5 : fl_lib/Electrical/Electrical Elements/Capacitor  c=Cgs nF  r=1e-12 Ohm  g=0 1/Ohm  i_specify=off  i_priority=None  i=0 A  i_nominal_specify=off  i_nominal_unit=A  i_nominal_value=1  v_specify=off  v_priority=None  v=0 V  v_nominal_specify=off  v_nominal_unit=V  v_nominal_value=1  vc_specify=off  vc_priority=High  vc=0 V  vc_nominal_specify=off  vc_nominal_unit=V  vc_nominal_value=1
  N-Type OFET : SimscapeComponentBlock  SourceFile=N_Marinov_OFET  ComponentPath=N_Marinov_OFET  ComponentVariants=N_Marinov_OFET  ComponentVariantNames=N_Marinov_OFET  ClassName=N_Marinov_OFET  SchemaVersion=1  Gamma=gama_n  Lambda=landa_n  Vbb=Vbb_n  Vss=Vss_n  aaa=aaa_n  bbb=bbb_n  ccc=ccc_n  Mu0=mu0_n  Vt=Vt_n V  Cox=ci  W=W_n  L=l  i_specify=off  i_priority=None  i=0 A  i_nominal_specify=off  i_nominal_unit=A  i_nominal_value=1  Vgs_specify=off  Vgs_priority=None  Vgs=0 V  Vgs_nominal_specify=off  Vgs_nominal_unit=V  Vgs_nominal_value=1  Vds_specify=off  Vds_priority=None  Vds=0 V  Vds_nominal_specify=off  Vds_nominal_unit=V  Vds_nominal_value=1  Power_specify=off  Power_priority=None  Power=0 W  Power_nominal_specify=off  Power_nominal_unit=W  Power_nominal_value=1
      settings: CopyFcn=simscape.engine.sli.internal.componentblockcallback(gcbh,'COPY')  PreCopyFcn=simscape.engine.sli.internal.componentblockcallback(gcbh,'PRECOPY')  PreDeleteFcn=simscape.engine.sli.internal.componentblockcallback(gcbh,'PREDELETE')  InternalSimscapePortConfiguration="{\"Bottom\":[],\"Left\":[{\"id\":\"g\",\"label\":\"Gate\",\"type\":\"foundation.electrical.electrical\"}],\"Right\":[{\"id\":\"d\",\"label\":\"Drain\",\"type\":\"foundation.electrical.electrical\"},{\"id\":\"s\",\"label\":\"Source\",\"type\":\"foundation.electrical.electrical\"}],\"Top\":[]}"
      mask Type: Marinov OFET
  P-Type OFET : SimscapeComponentBlock  SourceFile=P_Marinov_OFET  ComponentPath=P_Marinov_OFET  ComponentVariants=P_Marinov_OFET  ComponentVariantNames=P_Marinov_OFET  ClassName=P_Marinov_OFET  SchemaVersion=1  Gamma=gama_p  Lambda=landa_p  Vbb=Vbb_p  Vss=Vss_p  aaa=aaa_p  bbb=bbb_p  ccc=ccc_p  Mu0=mu0_p  Vt=Vt_p V  Cox=ci  W=W_p  L=l  i_specify=off  i_priority=None  i=0 A  i_nominal_specify=off  i_nominal_unit=A  i_nominal_value=1  Vsg_specify=off  Vsg_priority=None  Vsg=0 V  Vsg_nominal_specify=off  Vsg_nominal_unit=V  Vsg_nominal_value=1  Vsd_specify=off  Vsd_priority=None  Vsd=0 V  Vsd_nominal_specify=off  Vsd_nominal_unit=V  Vsd_nominal_value=1  Power_specify=off  Power_priority=None  Power=0 W  Power_nominal_specify=off  Power_nominal_unit=W  Power_nominal_value=1
      settings: CopyFcn=simscape.engine.sli.internal.componentblockcallback(gcbh,'COPY')  PreCopyFcn=simscape.engine.sli.internal.componentblockcallback(gcbh,'PRECOPY')  PreDeleteFcn=simscape.engine.sli.internal.componentblockcallback(gcbh,'PREDELETE')  InternalSimscapePortConfiguration="{\"Bottom\":[],\"Left\":[{\"id\":\"g\",\"label\":\"Gate\",\"type\":\"foundation.electrical.electrical\"}],\"Right\":[{\"id\":\"s\",\"label\":\"Source\",\"type\":\"foundation.electrical.electrical\"},{\"id\":\"d\",\"label\":\"Drain\",\"type\":\"foundation.electrical.electrical\"}],\"Top\":[]}"
      mask Type: Marinov OFET
  Probe1 : SimscapeProbe  BoundBlock=23  Variables={Power}
  Probe3 : SimscapeProbe  BoundBlock=24  Variables={Power}
  Scope1 : Scope
  Scope5 : Scope
  Input : PMIOPort  Side=Left
  Vdd : PMIOPort  Port=2  Side=Left
  Output : PMIOPort  Port=3  Side=Right
  Ground : PMIOPort  Port=4  Side=Left
  wires:
  Probe1/1 -> Scope1/1
  Probe3/1 -> Scope5/1
  connections:
  Vdd/RConn1 -- P-Type OFET/RConn1
  Ground/RConn1 -- Capacitor5/RConn1 -- N-Type OFET/RConn2
  P-Type OFET/LConn1 -- Input/RConn1 -- Capacitor5/LConn1 -- N-Type OFET/LConn1
  P-Type OFET/RConn2 -- N-Type OFET/RConn1 -- Output/RConn1

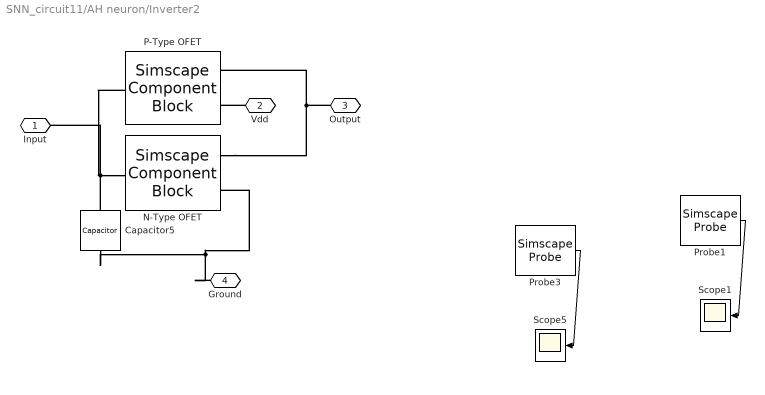
== system SNN_circuit11/AH neuron/Inverter2 ==
  Capacitor5 : fl_lib/Electrical/Electrical Elements/Capacitor  c=Cgs nF  r=1e-12 Ohm  g=0 1/Ohm  i_specify=off  i_priority=None  i=0 A  i_nominal_specify=off  i_nominal_unit=A  i_nominal_value=1  v_specify=off  v_priority=None  v=0 V  v_nominal_specify=off  v_nominal_unit=V  v_nominal_value=1  vc_specify=off  vc_priority=High  vc=0 V  vc_nominal_specify=off  vc_nominal_unit=V  vc_nominal_value=1
  N-Type OFET : SimscapeComponentBlock  SourceFile=N_Marinov_OFET  ComponentPath=N_Marinov_OFET  ComponentVariants=N_Marinov_OFET  ComponentVariantNames=N_Marinov_OFET  ClassName=N_Marinov_OFET  SchemaVersion=1  Gamma=gama_n  Lambda=landa_n  Vbb=Vbb_n  Vss=Vss_n  aaa=aaa_n  bbb=bbb_n  ccc=ccc_n  Mu0=mu0_n  Vt=Vt_n V  Cox=ci  W=W_n  L=l  i_specify=off  i_priority=None  i=0 A  i_nominal_specify=off  i_nominal_unit=A  i_nominal_value=1  Vgs_specify=off  Vgs_priority=None  Vgs=0 V  Vgs_nominal_specify=off  Vgs_nominal_unit=V  Vgs_nominal_value=1  Vds_specify=off  Vds_priority=None  Vds=0 V  Vds_nominal_specify=off  Vds_nominal_unit=V  Vds_nominal_value=1  Power_specify=off  Power_priority=None  Power=0 W  Power_nominal_specify=off  Power_nominal_unit=W  Power_nominal_value=1
      settings: CopyFcn=simscape.engine.sli.internal.componentblockcallback(gcbh,'COPY')  PreCopyFcn=simscape.engine.sli.internal.componentblockcallback(gcbh,'PRECOPY')  PreDeleteFcn=simscape.engine.sli.internal.componentblockcallback(gcbh,'PREDELETE')  InternalSimscapePortConfiguration="{\"Bottom\":[],\"Left\":[{\"id\":\"g\",\"label\":\"Gate\",\"type\":\"foundation.electrical.electrical\"}],\"Right\":[{\"id\":\"d\",\"label\":\"Drain\",\"type\":\"foundation.electrical.electrical\"},{\"id\":\"s\",\"label\":\"Source\",\"type\":\"foundation.electrical.electrical\"}],\"Top\":[]}"
      mask Type: Marinov OFET
  P-Type OFET : SimscapeComponentBlock  SourceFile=P_Marinov_OFET  ComponentPath=P_Marinov_OFET  ComponentVariants=P_Marinov_OFET  ComponentVariantNames=P_Marinov_OFET  ClassName=P_Marinov_OFET  SchemaVersion=1  Gamma=gama_p  Lambda=landa_p  Vbb=Vbb_p  Vss=Vss_p  aaa=aaa_p  bbb=bbb_p  ccc=ccc_p  Mu0=mu0_p  Vt=Vt_p V  Cox=ci  W=W_p  L=l  i_specify=off  i_priority=None  i=0 A  i_nominal_specify=off  i_nominal_unit=A  i_nominal_value=1  Vsg_specify=off  Vsg_priority=None  Vsg=0 V  Vsg_nominal_specify=off  Vsg_nominal_unit=V  Vsg_nominal_value=1  Vsd_specify=off  Vsd_priority=None  Vsd=0 V  Vsd_nominal_specify=off  Vsd_nominal_unit=V  Vsd_nominal_value=1  Power_specify=off  Power_priority=None  Power=0 W  Power_nominal_specify=off  Power_nominal_unit=W  Power_nominal_value=1
      settings: CopyFcn=simscape.engine.sli.internal.componentblockcallback(gcbh,'COPY')  PreCopyFcn=simscape.engine.sli.internal.componentblockcallback(gcbh,'PRECOPY')  PreDeleteFcn=simscape.engine.sli.internal.componentblockcallback(gcbh,'PREDELETE')  InternalSimscapePortConfiguration="{\"Bottom\":[],\"Left\":[{\"id\":\"g\",\"label\":\"Gate\",\"type\":\"foundation.electrical.electrical\"}],\"Right\":[{\"id\":\"s\",\"label\":\"Source\",\"type\":\"foundation.electrical.electrical\"},{\"id\":\"d\",\"label\":\"Drain\",\"type\":\"foundation.electrical.electrical\"}],\"Top\":[]}"
      mask Type: Marinov OFET
  Probe1 : SimscapeProbe  BoundBlock=30  Variables={Power}
  Probe3 : SimscapeProbe  BoundBlock=31  Variables={Power}
  Scope1 : Scope
  Scope5 : Scope
  Input : PMIOPort  Side=Left
  Vdd : PMIOPort  Port=2  Side=Left
  Output : PMIOPort  Port=3  Side=Right
  Ground : PMIOPort  Port=4  Side=Left
  wires:
  Probe1/1 -> Scope1/1
  Probe3/1 -> Scope5/1
  connections:
  N-Type OFET/RConn1 -- Output/RConn1 -- P-Type OFET/RConn2
  Input/RConn1 -- P-Type OFET/LConn1 -- Capacitor5/LConn1 -- N-Type OFET/LConn1
  Ground/RConn1 -- Capacitor5/RConn1 -- N-Type OFET/RConn2
  Vdd/RConn1 -- P-Type OFET/RConn1

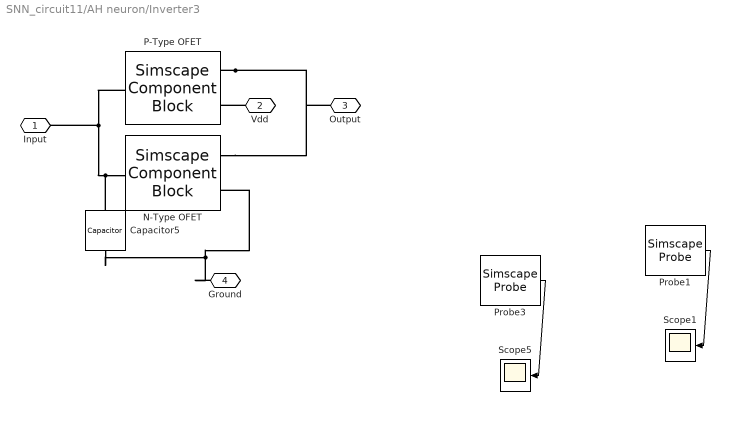
== system SNN_circuit11/AH neuron/Inverter3 ==
  Capacitor5 : fl_lib/Electrical/Electrical Elements/Capacitor  c=Cgs nF  r=1e-12 Ohm  g=0 1/Ohm  i_specify=off  i_priority=None  i=0 A  i_nominal_specify=off  i_nominal_unit=A  i_nominal_value=1  v_specify=off  v_priority=None  v=0 V  v_nominal_specify=off  v_nominal_unit=V  v_nominal_value=1  vc_specify=off  vc_priority=High  vc=0 V  vc_nominal_specify=off  vc_nominal_unit=V  vc_nominal_value=1
  N-Type OFET : SimscapeComponentBlock  SourceFile=N_Marinov_OFET  ComponentPath=N_Marinov_OFET  ComponentVariants=N_Marinov_OFET  ComponentVariantNames=N_Marinov_OFET  ClassName=N_Marinov_OFET  SchemaVersion=1  Gamma=gama_n  Lambda=landa_n  Vbb=Vbb_n  Vss=Vss_n  aaa=aaa_n  bbb=bbb_n  ccc=ccc_n  Mu0=mu0_n  Vt=Vt_n V  Cox=ci  W=W_n  L=l  i_specify=off  i_priority=None  i=0 A  i_nominal_specify=off  i_nominal_unit=A  i_nominal_value=1  Vgs_specify=off  Vgs_priority=None  Vgs=0 V  Vgs_nominal_specify=off  Vgs_nominal_unit=V  Vgs_nominal_value=1  Vds_specify=off  Vds_priority=None  Vds=0 V  Vds_nominal_specify=off  Vds_nominal_unit=V  Vds_nominal_value=1  Power_specify=off  Power_priority=None  Power=0 W  Power_nominal_specify=off  Power_nominal_unit=W  Power_nominal_value=1
      settings: CopyFcn=simscape.engine.sli.internal.componentblockcallback(gcbh,'COPY')  PreCopyFcn=simscape.engine.sli.internal.componentblockcallback(gcbh,'PRECOPY')  PreDeleteFcn=simscape.engine.sli.internal.componentblockcallback(gcbh,'PREDELETE')  InternalSimscapePortConfiguration="{\"Bottom\":[],\"Left\":[{\"id\":\"g\",\"label\":\"Gate\",\"type\":\"foundation.electrical.electrical\"}],\"Right\":[{\"id\":\"d\",\"label\":\"Drain\",\"type\":\"foundation.electrical.electrical\"},{\"id\":\"s\",\"label\":\"Source\",\"type\":\"foundation.electrical.electrical\"}],\"Top\":[]}"
      mask Type: Marinov OFET
  P-Type OFET : SimscapeComponentBlock  SourceFile=P_Marinov_OFET  ComponentPath=P_Marinov_OFET  ComponentVariants=P_Marinov_OFET  ComponentVariantNames=P_Marinov_OFET  ClassName=P_Marinov_OFET  SchemaVersion=1  Gamma=gama_p  Lambda=landa_p  Vbb=Vbb_p  Vss=Vss_p  aaa=aaa_p  bbb=bbb_p  ccc=ccc_p  Mu0=mu0_p  Vt=Vt_p V  Cox=ci  W=W_p  L=l  i_specify=off  i_priority=None  i=0 A  i_nominal_specify=off  i_nominal_unit=A  i_nominal_value=1  Vsg_specify=off  Vsg_priority=None  Vsg=0 V  Vsg_nominal_specify=off  Vsg_nominal_unit=V  Vsg_nominal_value=1  Vsd_specify=off  Vsd_priority=None  Vsd=0 V  Vsd_nominal_specify=off  Vsd_nominal_unit=V  Vsd_nominal_value=1  Power_specify=off  Power_priority=None  Power=0 W  Power_nominal_specify=off  Power_nominal_unit=W  Power_nominal_value=1
      settings: CopyFcn=simscape.engine.sli.internal.componentblockcallback(gcbh,'COPY')  PreCopyFcn=simscape.engine.sli.internal.componentblockcallback(gcbh,'PRECOPY')  PreDeleteFcn=simscape.engine.sli.internal.componentblockcallback(gcbh,'PREDELETE')  InternalSimscapePortConfiguration="{\"Bottom\":[],\"Left\":[{\"id\":\"g\",\"label\":\"Gate\",\"type\":\"foundation.electrical.electrical\"}],\"Right\":[{\"id\":\"s\",\"label\":\"Source\",\"type\":\"foundation.electrical.electrical\"},{\"id\":\"d\",\"label\":\"Drain\",\"type\":\"foundation.electrical.electrical\"}],\"Top\":[]}"
      mask Type: Marinov OFET
  Probe1 : SimscapeProbe  BoundBlock=37  Variables={Power}
  Probe3 : SimscapeProbe  BoundBlock=38  Variables={Power}
  Scope1 : Scope
  Scope5 : Scope
  Input : PMIOPort  Side=Left
  Vdd : PMIOPort  Port=2  Side=Left
  Output : PMIOPort  Port=3  Side=Right
  Ground : PMIOPort  Port=4  Side=Left
  wires:
  Probe1/1 -> Scope1/1
  Probe3/1 -> Scope5/1
  connections:
  Vdd/RConn1 -- P-Type OFET/RConn1
  Ground/RConn1 -- Capacitor5/RConn1 -- N-Type OFET/RConn2
  P-Type OFET/LConn1 -- Input/RConn1 -- Capacitor5/LConn1 -- N-Type OFET/LConn1
  P-Type OFET/RConn2 -- N-Type OFET/RConn1 -- Output/RConn1

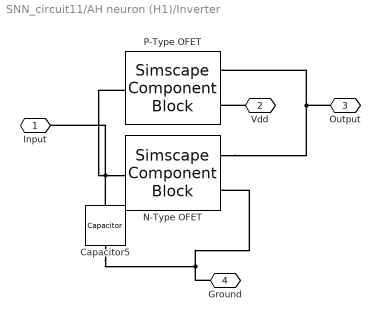
== system SNN_circuit11/AH neuron (H1)/Inverter ==
  Capacitor5 : fl_lib/Electrical/Electrical Elements/Capacitor  c=Cgs nF  r=1e-12 Ohm  g=0 1/Ohm  i_specify=off  i_priority=None  i=0 A  i_nominal_specify=off  i_nominal_unit=A  i_nominal_value=1  v_specify=off  v_priority=None  v=0 V  v_nominal_specify=off  v_nominal_unit=V  v_nominal_value=1  vc_specify=off  vc_priority=High  vc=0 V  vc_nominal_specify=off  vc_nominal_unit=V  vc_nominal_value=1
  N-Type OFET : SimscapeComponentBlock  SourceFile=N_Marinov_OFET  ComponentPath=N_Marinov_OFET  ComponentVariants=N_Marinov_OFET  ComponentVariantNames=N_Marinov_OFET  ClassName=N_Marinov_OFET  SchemaVersion=1  Gamma=gama_n  Lambda=landa_n  Vbb=Vbb_n  Vss=Vss_n  aaa=aaa_n  bbb=bbb_n  ccc=ccc_n  Mu0=mu0_n  Vt=Vt_n V  Cox=ci  W=W_n  L=l  i_specify=off  i_priority=None  i=0 A  i_nominal_specify=off  i_nominal_unit=A  i_nominal_value=1  Vgs_specify=off  Vgs_priority=None  Vgs=0 V  Vgs_nominal_specify=off  Vgs_nominal_unit=V  Vgs_nominal_value=1  Vds_specify=off  Vds_priority=None  Vds=0 V  Vds_nominal_specify=off  Vds_nominal_unit=V  Vds_nominal_value=1  Power_specify=off  Power_priority=None  Power=0 W  Power_nominal_specify=off  Power_nominal_unit=W  Power_nominal_value=1
      settings: CopyFcn=simscape.engine.sli.internal.componentblockcallback(gcbh,'COPY')  PreCopyFcn=simscape.engine.sli.internal.componentblockcallback(gcbh,'PRECOPY')  PreDeleteFcn=simscape.engine.sli.internal.componentblockcallback(gcbh,'PREDELETE')  InternalSimscapePortConfiguration="{\"Bottom\":[],\"Left\":[{\"id\":\"g\",\"label\":\"Gate\",\"type\":\"foundation.electrical.electrical\"}],\"Right\":[{\"id\":\"d\",\"label\":\"Drain\",\"type\":\"foundation.electrical.electrical\"},{\"id\":\"s\",\"label\":\"Source\",\"type\":\"foundation.electrical.electrical\"}],\"Top\":[]}"
      mask Type: Marinov OFET
  P-Type OFET : SimscapeComponentBlock  SourceFile=P_Marinov_OFET  ComponentPath=P_Marinov_OFET  ComponentVariants=P_Marinov_OFET  ComponentVariantNames=P_Marinov_OFET  ClassName=P_Marinov_OFET  SchemaVersion=1  Gamma=gama_p  Lambda=landa_p  Vbb=Vbb_p  Vss=Vss_p  aaa=aaa_p  bbb=bbb_p  ccc=ccc_p  Mu0=mu0_p  Vt=Vt_p V  Cox=ci  W=W_p  L=l  i_specify=off  i_priority=None  i=0 A  i_nominal_specify=off  i_nominal_unit=A  i_nominal_value=1  Vsg_specify=off  Vsg_priority=None  Vsg=0 V  Vsg_nominal_specify=off  Vsg_nominal_unit=V  Vsg_nominal_value=1  Vsd_specify=off  Vsd_priority=None  Vsd=0 V  Vsd_nominal_specify=off  Vsd_nominal_unit=V  Vsd_nominal_value=1  Power_specify=off  Power_priority=None  Power=0 W  Power_nominal_specify=off  Power_nominal_unit=W  Power_nominal_value=1
      settings: CopyFcn=simscape.engine.sli.internal.componentblockcallback(gcbh,'COPY')  PreCopyFcn=simscape.engine.sli.internal.componentblockcallback(gcbh,'PRECOPY')  PreDeleteFcn=simscape.engine.sli.internal.componentblockcallback(gcbh,'PREDELETE')  InternalSimscapePortConfiguration="{\"Bottom\":[],\"Left\":[{\"id\":\"g\",\"label\":\"Gate\",\"type\":\"foundation.electrical.electrical\"}],\"Right\":[{\"id\":\"s\",\"label\":\"Source\",\"type\":\"foundation.electrical.electrical\"},{\"id\":\"d\",\"label\":\"Drain\",\"type\":\"foundation.electrical.electrical\"}],\"Top\":[]}"
      mask Type: Marinov OFET
  Input : PMIOPort  Side=Left
  Vdd : PMIOPort  Port=2  Side=Left
  Output : PMIOPort  Port=3  Side=Right
  Ground : PMIOPort  Port=4  Side=Left
  connections:
  N-Type OFET/RConn1 -- Output/RConn1 -- P-Type OFET/RConn2
  Input/RConn1 -- P-Type OFET/LConn1 -- Capacitor5/LConn1 -- N-Type OFET/LConn1
  Ground/RConn1 -- N-Type OFET/RConn2 -- Capacitor5/RConn1
  Vdd/RConn1 -- P-Type OFET/RConn1
